simulink model "phase5_multibody"  (R2026a)
settings: Solver=VariableStepAuto
undefined symbols (not defined in the file): X, Y, Z
libraries: sm_lib x48, nesl_utility x39, fl_lib x30
(part 8 of 8)

== matlab function phase5_multibody/Pneumatic Leg 5/MATLAB Function1 ==
  data: x_dot input; z_dot output; z input
function z_dot = fcn(x_dot, z)
% Bouc-Wen Hysteresis parameters for soft silicone (n=1)
A = 1.0;
beta = 1.5;
gamma = 0.5;

% The Bouc-Wen differential equation
z_dot = A * x_dot - beta * abs(x_dot) * z - gamma * x_dot * abs(z);
end

== matlab function phase5_multibody/Pneumatic Leg 6/MATLAB Function1 ==
  data: x_dot input; z_dot output; z input
function z_dot = fcn(x_dot, z)
% Bouc-Wen Hysteresis parameters for soft silicone (n=1)
A = 1.0;
beta = 1.5;
gamma = 0.5;

% The Bouc-Wen differential equation
z_dot = A * x_dot - beta * abs(x_dot) * z - gamma * x_dot * abs(z);
end

== matlab function phase5_multibody/Pneumatic Leg 4/MATLAB Function1 ==
  data: x_dot input; z_dot output; z input
function z_dot = fcn(x_dot, z)
% Bouc-Wen Hysteresis parameters for soft silicone (n=1)
A = 1.0;
beta = 1.5;
gamma = 0.5;

% The Bouc-Wen differential equation
z_dot = A * x_dot - beta * abs(x_dot) * z - gamma * x_dot * abs(z);
end

== matlab function phase5_multibody/Pneumatic Leg 2/MATLAB Function1 ==
  data: x_dot input; z_dot output; z input
function z_dot = fcn(x_dot, z)
% Bouc-Wen Hysteresis parameters for soft silicone (n=1)
A = 1.0;
beta = 1.5;
gamma = 0.5;

% The Bouc-Wen differential equation
z_dot = A * x_dot - beta * abs(x_dot) * z - gamma * x_dot * abs(z);
end

== matlab function phase5_multibody/Pneumatic Leg 3/MATLAB Function1 ==
  data: x_dot input; z_dot output; z input
function z_dot = fcn(x_dot, z)
% Bouc-Wen Hysteresis parameters for soft silicone (n=1)
A = 1.0;
beta = 1.5;
gamma = 0.5;

% The Bouc-Wen differential equation
z_dot = A * x_dot - beta * abs(x_dot) * z - gamma * x_dot * abs(z);
end

== matlab function phase5_multibody/Pneumatic Leg 1/MATLAB Function1 ==
  data: x_dot input; z_dot output; z input
function z_dot = fcn(x_dot, z)
% Bouc-Wen Hysteresis parameters for soft silicone (n=1)
A = 1.0;
beta = 1.5;
gamma = 0.5;

% The Bouc-Wen differential equation
z_dot = A * x_dot - beta * abs(x_dot) * z - gamma * x_dot * abs(z);
end
